simulink model "arducopter"  (R2021a)
settings: Solver=FixedStepAuto  StartTime=0.0  StopTime=sim.param.timeEnd  FixedStep=sim.param.dt  RelTol=1e-3
undefined symbols (not defined in the file or in its folder): DiscIntNeverNeededParam, sim
libraries: simulink x34, slident x4, vrlib x1
(part 7 of 8)

== matlab function arducopter/Position Controller/P Position z/Set vertical speed & acceleration limit/Set error limits ==
function [errMin, errMax, D1max] = setLimits(outMin, outMax, DoutMax, D2OutMax, kp)
% Code taken from AC_P_1D::set_limits() in AC_P_1D.cpp.
% Input parameter D2_out_max is neglected since it is set to zero in
% AC_PosControl::set_correction_speed_accel_z()

errMin = single(0.0);
errMax = single(0.0);
D1max = single(0.0);

if (DoutMax > 0)
   D1max = DoutMax; 
end

% Missing line left out because of parameter D2_out_max being set to 0

% Call the simulink function inv_sqrt_controller(...) from control.cpp,
% line 343 if the conditions apply
if (outMin < 0 && kp > 0)
    errMin = inv_sqrt_controller(outMin, kp, DoutMax);
end

if (outMax > 0 && kp > 0)
    errMax = inv_sqrt_controller(outMax, kp, DoutMax);
end

== matlab function arducopter/Position Controller/P Position z/Set vertical speed & acceleration limit/Inverse Square Root Controller/Inverse Sqrt Controller ==
function errLim = inv_sqrt_controller(output, p, Dmax)
% Code taken from inv_sqrt_controller(...) in control.cpp.
% Function calculates the input (error) to the sqrt_controller required to
% achieve a given output

if (Dmax > 0 && p == 0)
    errLim = output * output / (single(2.0) * Dmax);
    return;
end
if ((Dmax < 0 || Dmax == 0) && p ~= 0)
    errLim = output / p;
    return;
end
if ((Dmax < 0 || Dmax == 0) && p == 0)
   errLim = single(0.0);
   return
end

% Calculate the cross-point velocity, at which we switch from calculating the
% controller output using a linear function to a sqrt function
linear_velocity = Dmax / p;
% Use linear function to calculate limit if current velocity is below
% cross-point velocity
if (abs(output) < linear_velocity)
   errLim = output / p;
   return;
end

% Calculate the cross-point distance at which we switch to sqrt function
linear_dist = Dmax / (p*p);
% Calculate the maximum distance error resulting from the velocity and
% acceleration limit
stopping_dist = (linear_dist * single(0.5)) + (output*output) / (single(2.0) * Dmax);
% If output parameter is negative or zero, return negative maximum distance
% error
if (output > 0)
    errLim = stopping_dist;
else
    errLim = -stopping_dist;
end

== matlab function arducopter/Position Controller/P Position z/Square Root Controller ==
function correction_rate = sqrt_controller(err, p, second_ord_lim, dt)
% The square root controller
% Code is taken from sqrt_controller(...) in AC_PosControl.cpp.

if (second_ord_lim < 0 || second_ord_lim == 0)
   correction_rate = err * p;
elseif (p == 0)
    % P term is zero, but second order limit is positive
    if (err > 0)
        correction_rate = sqrt(single(2.0) * second_ord_lim * err);
    elseif (err < 0)
        correction_rate = sqrt(single(2.0) * second_ord_lim * -err);
    else
        correction_rate = single(0.0);
    end
else
    % P term and second order limit are positive, hence have been defined
    linear_dist = second_ord_lim / (p * p);
    % Check if error exceeds linear range of controller gain
    if (err > linear_dist)
        correction_rate = sqrt(single(2.0) * second_ord_lim * ( err - (linear_dist / single(2.0)) ));
    elseif (err < -linear_dist)
        correction_rate = -sqrt(single(2.0) * second_ord_lim * ( -err - (linear_dist / single(2.0)) ));
    else
        % Return linearly amplified correction if error is in linear range
        correction_rate = err * p;
    end
end

% Prevent oscillations by over-shooting the error correction in the last
% time step
if (dt ~= 0)
    correction_rate = max( min(correction_rate, abs(err) / dt), -abs(err) / dt);
end

== matlab function arducopter/Position Controller/PID Acceleration z/Slew Limiter/Lowpass Filter ==
function out  = fcn(in, cutoff_freq, loop_rate, out_last)
% The code is based on the apply(sample, cutoff_freq, dt) function in
% LowPassFilter.cpp
dt = 1 / loop_rate;

% Check if filter is supposed to be filtering
if (cutoff_freq <=0 || dt <= 0)
    out = in;
    return;
end

% Calculate time constant and alpha value
T = 1 / (2 * pi * cutoff_freq);
alpha = dt / (dt + T);
alpha = max( min( alpha, 1.0), 0.0);

% Output calculation
out = out_last + (in - out_last) * alpha;

== matlab function arducopter/Throttle/Throttle Calculations/Throttle-Attitude-Mixing/Update Throttle Mix Des ==
function thrMixDes = updateThrottleMix(thrTar, zVelCtrlRatio, zVelDes, thrMan, thrMixMin, thrMixMax, thrMixMan)
% Sets desired throttle vs attitude priorization based on vehicle state.
% Low values favour pilot/autpilot throttle over attitude control, high
% values favour attitude control over throttle
% Has not effec twhen throttle > hover throttle
% Code: land_detector.cpp, Copter::update_throttle_mix()

if thrMan
    % Manual throttle
    if thrTar <= 0
        % Call to set_throttle_mix_min() set mix to minimum
        thrMixDes = thrMixMin;
    else
        % Call to set_throttle_mix_man() sets mix to value for manual
        % throttle
        thrMixDes = thrMixMan;
    end
else
    % Autopilot controlled throttle
    
    % Check for aggressive flight request - Requested roll/pitch angle
    % above 15 degrees
    % ToDo

    % Check for large external disturbances - angle error over 30 degrees
    % ToDo

    % Check for large acceleration - falling for high turbulence
    % ToDo

    % Check for requested descent
    descent_not_demanded = zVelDes >= single(0.0);

    if (descent_not_demanded)
        % Call to AC_AttitudeControl_Multi::set_throttle_mix_max(ratio)
        ratio = min( max(single(0.0), zVelCtrlRatio), single(1.0) );
        thrMixDes = (single(1.0) - ratio) * thrMixMin + ratio * thrMixMax;
    else
        thrMixDes = thrMixMin;
    end
end

== matlab function arducopter/Position Controller/zVelCtrlRatio Calculation/Update vel_z_ctrl_ratio ==
function zVelCtrlRat = setZVelCtrlRatio(velErr, dnVelMax, dt)
% Sets vel_z_control_ratio, which contains the proportion of the z velocity
% error relative to the maximum request. Needed in function
% Copter::update_throttle_mix().
% Code: AC_PosControl.cpp, update_z_controller()

global vel_z_ctrl_ratio;

err_ratio = velErr / dnVelMax;
vel_z_ctrl_ratio = vel_z_ctrl_ratio + dt * single(0.1) * (0.5 - err_ratio);
vel_z_ctrl_ratio = min( max(single(0.0), vel_z_ctrl_ratio), single(2.0) );

zVelCtrlRat = vel_z_ctrl_ratio;

== matlab function arducopter/Position Controller/Vertical Speed and Acceleration Limits ==
function setMaxSpeedAccelZ(dnSpeedMax, upSpeedMax, zAccMax, zJerkMax, GRAVITY_MSS, zAccFltt_f, zAccFlte_f)
% Sets the maximum vertical speed in cm/s and acceleration in cm/s/s.
% Checks max vertical jerk limits.
% Code: AC_PosControl.cpp, set_max_speed_accel_z().

global vel_max_down_cms;
global vel_max_up_cms;
global acc_max_z_cmss;
global jerk_max_z_cmsss;

% Make sure maximum descending speed is negative
dnSpeedMax = dnSpeedMax * single(-1);

% Sanity check
if dnSpeedMax < 0
    vel_max_down_cms = dnSpeedMax;
end
if upSpeedMax > 0
    vel_max_up_cms = upSpeedMax;
end
if zAccMax > 0
    acc_max_z_cmss = zAccMax;
end

% Ensure that vertical jerk is not limited by filter of z acceleration PID
jerk_max_z_cmsss = single(100) * zJerkMax;
if (zAccFltt_f > 0)
    jerk_max_z_cmsss = min( jerk_max_z_cmsss, min(GRAVITY_MSS * single(100), acc_max_z_cmss) * (2*pi*zAccFltt_f) / single(5.0) );
end
if (zAccFlte_f > 0)
    jerk_max_z_cmsss = min( jerk_max_z_cmsss, min(GRAVITY_MSS * single(100), acc_max_z_cmss) * (2*pi*zAccFlte_f) / single(5.0) );
end

== matlab function arducopter/Lowpass2p/Lowpass Pitch/Lowpass2p ==
function y = lowpass2p(u, sampleFreq, cutoffFreq)
% Lowpass filter of order two
% Source: LowPassFilter2p.cpp
global delElem1
global delElem2

% Calculate parameters: LowPassFilter2p.cpp, compute_params()
fr = single(sampleFreq/cutoffFreq);
ohm = single(tan(pi/fr));
c = single(1+2*cos(pi/4)*ohm + ohm*ohm);

b0 = ohm*ohm/c;
b1 = 2*b0;
b2 = b0;
a1 = 2*(ohm*ohm-1)/c;
a2 = single((1-2*cos(pi/4)*ohm+ohm*ohm)/c);

% Calculation of filtered sample: LowPassFilter2p.cpp, apply()
delElem0 = u - delElem1 * a1 - delElem2 * a2;
y = delElem0 * b0 + delElem1 * b1 + delElem2 * b2;

delElem2 = delElem1;
delElem1 = delElem0;

== matlab function arducopter/Lowpass2p/Lowpass Roll/Lowpass2p ==
function y = lowpass2p(u, sampleFreq, cutoffFreq)
% Lowpass filter of order two
% Source: LowPassFilter2p.cpp
global delElem1
global delElem2

% Calculate parameters: LowPassFilter2p.cpp, compute_params()
fr = single(sampleFreq/cutoffFreq);
ohm = single(tan(pi/fr));
c = single(1+2*cos(pi/4)*ohm + ohm*ohm);

b0 = ohm*ohm/c;
b1 = 2*b0;
b2 = b0;
a1 = 2*(ohm*ohm-1)/c;
a2 = single((1-2*cos(pi/4)*ohm+ohm*ohm)/c);

% Calculation of filtered sample: LowPassFilter2p.cpp, apply()
delElem0 = u - delElem1 * a1 - delElem2 * a2;
y = delElem0 * b0 + delElem1 * b1 + delElem2 * b2;

delElem2 = delElem1;
delElem1 = delElem0;

== matlab function arducopter/Lowpass2p/Lowpass Yaw/Lowpass2p ==
function y = lowpass2p(u, sampleFreq, cutoffFreq)
% Lowpass filter of order two
% Source: LowPassFilter2p.cpp
global delElem1
global delElem2

% Calculate parameters: LowPassFilter2p.cpp, compute_params()
fr = single(sampleFreq/cutoffFreq);
ohm = single(tan(pi/fr));
c = single(1+2*cos(pi/4)*ohm + ohm*ohm);

b0 = ohm*ohm/c;
b1 = 2*b0;
b2 = b0;
a1 = 2*(ohm*ohm-1)/c;
a2 = single((1-2*cos(pi/4)*ohm+ohm*ohm)/c);

% Calculation of filtered sample: LowPassFilter2p.cpp, apply()
delElem0 = u - delElem1 * a1 - delElem2 * a2;
y = delElem0 * b0 + delElem1 * b1 + delElem2 * b2;

delElem2 = delElem1;
delElem1 = delElem0;

== matlab function arducopter/Body Frame Rates -> DCM/MATLAB Function ==
function quaternion = from_rotation_matrix(dcm)
% Function to calculate quaternion from a given rotation matrix.
% Implemented based on QuaternionT<T>::from_rotation_matrx()

m00 = dcm(1,1);
m11 = dcm(2,2);
m22 = dcm(3,3);
m10 = dcm(2,1);
m01 = dcm(1,2);
m20 = dcm(3,1);
m02 = dcm(1,3);
m21 = dcm(3,2);
m12 = dcm(2,3);

tr = m00 + m11 + m22;

if tr > 0
    S = sqrt(tr+1) * 2;
    qw = 0.25 * S;
    qx = (m21 - m12) / S;
    qy = (m02 - m20) / S;
    qz = (m10 - m01) / S;
elseif ((m00 > m11) && (m00 > m22))
    S = sqrt(1.0 + m00 - m11 - m22) * 2.0;
    qw = (m21 - m12) / S;
    qx = 0.25 * S;
    qy = (m01 + m10) / S;
    qz = (m02 + m20) / S;
elseif (m11 > m22)
    S = sqrt(1.0 + m11 - m00 - m22) * 2.0;
    qw = (m02 - m20) / S;
    qx = (m01 + m10) / S;
    qy = 0.25 * S;
    qz = (m12 + m21) / S;
else
    S = sqrt(1.0 + m22 - m00 - m11) * 2.0;
    qw = (m10 - m01) / S;
    qx = (m02 + m20) / S;
    qy = (m12 + m21) / S;
    qz = 0.25 * S;
end

quaternion = [qw;qx;qy;qz];

== matlab function arducopter/Attitude Controller/MATLAB Function ==
function [rollOut, pitchOut] = get_pilot_desired_lean_angles(rollIn, pitchIn, angleMax, angleLimit)
% Code based on Mode::get_pilot_desired_lean_angles()
% Transform pilot's roll and pitch input into desired lean angle

% Limit max lean angle
angleLimit = max(min(angleLimit, angleMax), 1000);

% Scale roll and pitch inputs to ANGLE_MAX parameter range
scaler = angleMax / 4500; % 4500 is the default of ROLL_PITCH_YAW_INPUT_MAX
rollOut = rollIn * scaler;
pitchOut = pitchIn * scaler;

% Circular limit
quadNorm = sqrt(rollOut^2 + pitchOut^2);
if quadNorm > angleLimit
    ratio = angleLimit / quadNorm;
    rollOut = rollOut * ratio;
    pitchOut = pitchOut * ratio;
end

% Lateral tilt to euler roll conversion
rollOut = (18000/pi) * atan(cos(pitchOut*(pi/18000))*tan(rollOut*(pi/18000)));

== matlab function arducopter/Attitude Controller/MATLAB Function1 ==
function yawOut = get_pilot_desired_yaw_rate(yawIn, pilotYawExpo, pilotYawRate)
% Code taken from Mode::get_pilot_desired_yaw_rate()
% Transforms pilot's yaw input into a desired yaw rate

%% 1) Apply expo - Code based on input_expo in control.cpp
yawIn = min(max(yawIn, -1), 1);
if pilotYawExpo < 0.95
    yawIn = (1 - pilotYawExpo) * yawIn / (1 - pilotYawExpo * abs(yawIn));
end

%% 2) Convert pilot input to the desired yaw rate
yawOut = pilotYawRate * 100 * yawIn;

== matlab function arducopter/Attitude Controller/input_euler_angle_roll_pitch_euler_rate_yaw()/MATLAB Function ==
function [roll, pitch, yaw] = toEuler(q)
% Function takes a quaternion and translates it into Euler angles
% Based on QuaternionT<T>::to_euler() and incorporates 
% QuaternionT<T>::get_euler_roll(), QuaternionT<T>::get_euler_pitch() and
% QuaternionT<T>::get_euler_yaw()

roll = single(atan2(2 * (q(1)*q(2) + q(3)*q(4)), 1 - 2*(q(2)*q(2) + q(3)*q(3))));
% Check if argument of asin is greater than 1 oder smaller than -1
% Based on safe_asin() in AP_MATH.cpp
xPitch = 2 * (q(1)*q(3) - q(4)*q(2));
if xPitch >= 1
    pitch = single(pi/2);
elseif xPitch <= -1
    pitch = single(-pi/2);
else
    pitch = single(asin(xPitch));
end
yaw = single(atan2(2*(q(1)*q(4) + q(2)*q(3)), 1 - 2*(q(3)*q(3) + q(4)*q(4))));

== matlab function arducopter/Attitude Controller/input_euler_angle_roll_pitch_euler_rate_yaw()/Feedforward enabled/MATLAB Function ==
function eulerAccelMaxBF = euler_accel_limit(eulerAngleTar, eulerAccelMaxEF)
% Translation of acceleration limits eulerAccelMax to the euler axis
% Code based on AC_AttitudeControl::euler_accel_limit()

sin_phi = max(min(abs(single(sin(eulerAngleTar(1)))), 1), 0.1); % Sinus of roll angle
cos_phi = max(min(abs(single(cos(eulerAngleTar(1)))), 1), 0.1);
sin_theta = max(min(abs(single(sin(eulerAngleTar(2)))), 1), 0.1); % Sinus of pitch angle

eulerAccelMaxBF = single(zeros(3,1));
if eulerAccelMaxEF(1) == 0 || eulerAccelMaxEF(2) == 0 || eulerAccelMaxEF(3) == 0 || ...
   eulerAccelMaxEF(1) < 0 || eulerAccelMaxEF(2) < 0 || eulerAccelMaxEF(3) < 0 
    eulerAccelMaxBF(1) = eulerAccelMaxEF(1);
    eulerAccelMaxBF(2) = eulerAccelMaxEF(2);
    eulerAccelMaxBF(3) = eulerAccelMaxEF(3);
else
    eulerAccelMaxBF(1) = eulerAccelMaxEF(1);
    eulerAccelMaxBF(2) = min(eulerAccelMaxEF(2) / cos_phi, eulerAccelMaxEF(3) / sin_phi);
    eulerAccelMaxBF(3) = min(min(eulerAccelMaxEF(1) / sin_theta, eulerAccelMaxEF(2) / sin_phi), eulerAccelMaxEF(3) / cos_phi);
end

== matlab function arducopter/Attitude Controller/input_euler_angle_roll_pitch_euler_rate_yaw()/Feedforward enabled/input shaping/input shaping roll angle/Square Root Controller ==
function correction_rate = sqrt_controller(err, p, second_ord_lim, dt)
% The square root controller
% Code is taken from sqrt_controller(...) in AC_PosControl.cpp, line 296.

if (second_ord_lim < 0 || second_ord_lim == 0)
   correction_rate = err * p;
elseif (p == 0)
    % P term is zero, but second order limit is positive
    if (err > 0)
        correction_rate = sqrt(single(2.0) * second_ord_lim * err);
    elseif (err < 0)
        correction_rate = sqrt(single(2.0) * second_ord_lim * -err);
    else
        correction_rate = single(0.0);
    end
else
    % P term and second order limit are positive, hence have been defined
    linear_dist = second_ord_lim / (p * p);
    % Check if error exceeds linear range of controller gain
    if (err > linear_dist)
        correction_rate = sqrt(single(2.0) * second_ord_lim * ( err - (linear_dist / single(2.0)) ));
    elseif (err < -linear_dist)
        correction_rate = -sqrt(single(2.0) * second_ord_lim * ( -err - (linear_dist / single(2.0)) ));
    else
        % Return linearly amplified correction if error is in linear range
        correction_rate = err * p;
    end
end

% Prevent oscillations by over-shooting the error correction in the last
% time step
if (dt ~= 0)
    correction_rate = max( min(correction_rate, abs(err) / dt), -abs(err) / dt);
end

== matlab function arducopter/Attitude Controller/input_euler_angle_roll_pitch_euler_rate_yaw()/Feedforward enabled/input shaping/input shaping roll angle/MATLAB Function ==
function radLim = wrapPi(radIn)
% Function to limit input angle in radian to [-pi pi].
% Code based on wrap_PI() and wrap_2PI() of AP_Math.cpp

% 1) Limit to [0 2pi]
radLim = mod(radIn, 2*pi);
if radLim < 0
    radLim = radLim + 2*pi;
end

% 2) Limit to [0 pi]
if radLim > pi
    radLim = radLim - 2*pi;
end

== matlab function arducopter/Attitude Controller/input_euler_angle_roll_pitch_euler_rate_yaw()/Feedforward enabled/input shaping/input shaping roll angle/MATLAB Function1 ==
function eulerRateTar = input_shaping_ang_vel(desiredAngVel, targetAngVel, accelMax, dt)
% Limits acceleration and deceleration of a velocity request
% Code based on AC_AttitudeControl::input_shaping_ang_vel()

% Acceleration is limited directly to smooth the beginning of the curve
if accelMax > 0
    deltaAngVel = accelMax * dt;
    eulerRateTar = min(max(desiredAngVel, targetAngVel - deltaAngVel), targetAngVel + deltaAngVel);
else
    eulerRateTar = desiredAngVel;
end

== matlab function arducopter/Attitude Controller/input_euler_angle_roll_pitch_euler_rate_yaw()/Feedforward enabled/input shaping/input shaping pitch angle/MATLAB Function ==
function radLim = wrapPi(radIn)
% Function to limit input angle in radian to [-pi pi].
% Code based on wrap_PI() and wrap_2PI() of AP_Math.cpp

% 1) Limit to [0 2pi]
radLim = mod(radIn, 2*pi);
if radLim < 0
    radLim = radLim + 2*pi;
end

% 2) Limit to [0 pi]
if radLim > pi
    radLim = radLim - 2*pi;
end

== matlab function arducopter/Attitude Controller/input_euler_angle_roll_pitch_euler_rate_yaw()/reset yaw targets/MATLAB Function9 ==
function qRes = quatMult(q1, q2)
% Quaternion multiplication. Code based on QuaternionT<T>::operator*() in
% quaternion.cpp

qRes = single(zeros(4,1));
qRes(1) = q1(1)*q2(1) - q1(2)*q2(2) - q1(3)*q2(3) - q1(4)*q2(4);
qRes(2) = q1(1)*q2(2) + q1(2)*q2(1) + q1(3)*q2(4) - q1(4)*q2(3);
qRes(3) = q1(1)*q2(3) - q1(2)*q2(4) + q1(3)*q2(1) + q1(4)*q2(2);
qRes(4) = q1(1)*q2(4) + q1(2)*q2(3) - q1(3)*q2(2) + q1(4)*q2(1);

== matlab function arducopter/Attitude Controller/input_euler_angle_roll_pitch_euler_rate_yaw()/Feedforward enabled/input shaping/input shaping pitch angle/Square Root Controller ==
function correction_rate = sqrt_controller(err, p, second_ord_lim, dt)
% The square root controller
% Code is taken from sqrt_controller(...) in AC_PosControl.cpp, line 296.

if (second_ord_lim < 0 || second_ord_lim == 0)
   correction_rate = err * p;
elseif (p == 0)
    % P term is zero, but second order limit is positive
    if (err > 0)
        correction_rate = sqrt(single(2.0) * second_ord_lim * err);
    elseif (err < 0)
        correction_rate = sqrt(single(2.0) * second_ord_lim * -err);
    else
        correction_rate = single(0.0);
    end
else
    % P term and second order limit are positive, hence have been defined
    linear_dist = second_ord_lim / (p * p);
    % Check if error exceeds linear range of controller gain
    if (err > linear_dist)
        correction_rate = sqrt(single(2.0) * second_ord_lim * ( err - (linear_dist / single(2.0)) ));
    elseif (err < -linear_dist)
        correction_rate = -sqrt(single(2.0) * second_ord_lim * ( -err - (linear_dist / single(2.0)) ));
    else
        % Return linearly amplified correction if error is in linear range
        correction_rate = err * p;
    end
end

% Prevent oscillations by over-shooting the error correction in the last
% time step
if (dt ~= 0)
    correction_rate = max( min(correction_rate, abs(err) / dt), -abs(err) / dt);
end

== matlab function arducopter/Attitude Controller/input_euler_angle_roll_pitch_euler_rate_yaw()/Feedforward enabled/MATLAB Function1 ==
function angVelTar = euler_rate_to_ang_vel(eulerAngle, eulerRate)
% This function converts euler angle derivatives (321 system) to an angular
% velocity vector. eulerAngle is the vector of the euler angles in rad and
% eulerRate is the vector of euler rates in rad/s
% Code based on AC_AttitudeControl::euler_rate_to_ang_vel()

sin_theta = single(sin(eulerAngle(2)));
cos_theta = single(cos(eulerAngle(2)));
sin_phi = single(sin(eulerAngle(1)));
cos_phi = single(cos(eulerAngle(1)));

angVelTar = single(zeros(3,1));
angVelTar(1) = eulerRate(1) - sin_theta * eulerRate(3);
angVelTar(2) = cos_phi * eulerRate(2) + sin_phi * cos_theta * eulerRate(3);
angVelTar(3) = -sin_phi * eulerRate(2) + cos_theta * cos_phi * eulerRate(3);

== matlab function arducopter/Rate Controller/PID Pitch Rate/I/Integrator ==
function integrator_out = fcn(error, integrator, limit_flg, ki, i_max, dt)
% Code is based on AC_PID::update_i() in AC_PID.cpp.

% Check plausibility of input parameters
if (ki ~= 0 && dt > 0)
    % Only allow integration if limit is not set or the absolute sum of the
    % integrator would be reduced.
    if (~limit_flg || (integrator > 0 && error < 0) || (integrator < 0 && error > 0))
        integrator_out = integrator + error * ki * dt;
        integrator_out = max( min(integrator_out, i_max), -i_max);
    else % Otherwise, keep old integrator value
        integrator_out = integrator;
    end
else % Reset integrator if input parameters are not plausible
    integrator_out = single(0.0);
end

== matlab function arducopter/Attitude Controller/input_euler_angle_roll_pitch_euler_rate_yaw()/reset yaw targets/MATLAB Function1 ==
function [roll, pitch, yaw] = toEuler(q)
% Function takes a quaternion and translates it into Euler angles
% Based on QuaternionT<T>::to_euler() and incorporates 
% QuaternionT<T>::get_euler_roll(), QuaternionT<T>::get_euler_pitch() and
% QuaternionT<T>::get_euler_yaw()

roll = single(atan2(2 * (q(1)*q(2) + q(3)*q(4)), 1 - 2*(q(2)*q(2) + q(3)*q(3))));
% Check if argument of asin is greater than 1 oder smaller than -1
% Based on safe_asin() in AP_MATH.cpp
xPitch = 2 * (q(1)*q(3) - q(4)*q(2));
if xPitch >= 1
    pitch = single(pi/2);
elseif xPitch <= -1
    pitch = single(-pi/2);
else
    pitch = single(asin(xPitch));
end
yaw = single(atan2(2*(q(1)*q(4) + q(2)*q(3)), 1 - 2*(q(3)*q(3) + q(4)*q(4))));

== matlab function arducopter/Attitude Controller/input_euler_angle_roll_pitch_euler_rate_yaw()/Feedforward enabled/MATLAB Function2 ==
function angVelTarLimited = ang_vel_limit(angVelTar, angVelRollMax, angVelPitchMax, angVelYawMax)
% Limits angular velocity (rad/s) in body frame
% Code based on AC_AttitudeControl::ang_vel_limit()

angVelTarLimited = angVelTar;
if angVelRollMax == 0 || angVelPitchMax == 0
    if angVelRollMax ~= 0
        angVelTarLimited(1) = max(min(angVelTar(1), angVelRollMax), -angVelRollMax);
    end
    if angVelPitchMax ~= 0
        angVelTarLimited(2) = max(min(angVelTar(2), angVelPitchMax), -angVelPitchMax);
    end
else
    thrustVecAngVel = [angVelTar(1) / angVelRollMax; angVelTar(2) / angVelPitchMax];
    thrustVecLen = single(sqrt(thrustVecAngVel(1)^2 + thrustVecAngVel(2)^2));
    if thrustVecLen > 1
        angVelTarLimited(1) = thrustVecAngVel(1) * angVelRollMax / thrustVecLen;
        angVelTarLimited(2) = thrustVecAngVel(2) * angVelPitchMax / thrustVecLen;
    end
end
if angVelYawMax ~= 0
    angVelTarLimited(3) = max(min(angVelTar(3), angVelYawMax), -angVelYawMax);
end

== matlab function arducopter/Attitude Controller/input_euler_angle_roll_pitch_euler_rate_yaw()/Feedforward enabled/MATLAB Function3 ==
function eulerRate = ang_vel_to_euler_rate(angVelBf,eulerAngle)
% Function converts body-frame angular velocity into euler rate of desired
% attitude
% Based on AC_AttitudeControl::ang_vel_to_euler_rate()

sin_theta = single(sin(eulerAngle(2)));
cos_theta = single(cos(eulerAngle(2)));
sin_phi = single(sin(eulerAngle(1)));
cos_phi = single(cos(eulerAngle(1)));

eulerRate = single(zeros(3,1));
eulerRate(1) = angVelBf(1) + sin_phi * (sin_theta / cos_theta) * angVelBf(2) + cos_phi * (sin_theta / cos_theta) * angVelBf(3);
eulerRate(2) = cos_phi * angVelBf(2) - sin_phi * angVelBf(3);
eulerRate(3) = (sin_phi / cos_theta) * angVelBf(2) + (cos_phi / cos_theta) * angVelBf(3);

== matlab function arducopter/Attitude Controller/input_euler_angle_roll_pitch_euler_rate_yaw()/Feedforward disabled/MATLAB Function ==
function q = fromEuler(roll, pitch, yaw)
% Computes quaternion from euler angle vector
% Based on QuaternionT<T>::from_euler()

q = single(zeros(4,1));
cr2 = single(cos(roll*0.5));
cp2 = single(cos(pitch*0.5));
cy2 = single(cos(yaw*0.5));
sr2 = single(sin(roll*0.5));
sp2 = single(sin(pitch*0.5));
sy2 = single(sin(yaw*0.5));

q(1) = cr2*cp2*cy2 + sr2*sp2*sy2;
q(2) = sr2*cp2*cy2 - cr2*sp2*sy2;
q(3) = cr2*sp2*cy2 + sr2*cp2*sy2;
q(4) = cr2*cp2*sy2 - sr2*sp2*cy2;

== matlab function arducopter/Attitude Controller/input_euler_angle_roll_pitch_euler_rate_yaw()/thrust_heading_rotation_angles()/thrust_vector_rotation_angles()/MATLAB Function ==
function vecRot = rotateByQuat(q, vec)
% Function rotates vector vec by quaternion q. Equivalent to converting the
% input quaternion to a rotation matrix and then multiplying it by the
% vector. This uses the formula
%
%    v2 = v1 + 2 q1 * qv x v1 + 2 qv x qv x v1
%
% where "x" is the cross product (explicitly inlined for performance below), 
% "q1" is the scalar part and "qv" is the vector part of this quaternion
% Code based on Vector3<T> QuaternionT<T>::operator*()

vecRot = vec;

% Compute and cache "qv x v1"
uv = [q(3) * vec(3) - q(4) * vec(2); q(4) * vec(1) - q(2) * vec(3); q(2) * vec(2) - q(3) * vec(1)];

uv(1) = uv(1) + uv(1);
uv(2) = uv(2) + uv(2);
uv(3) = uv(3) + uv(3);
vecRot(1) = vecRot(1) + q(1) * uv(1) + q(3) * uv(3) - q(4) * uv(2);
vecRot(2) = vecRot(2) + q(1) * uv(2) + q(4) * uv(1) - q(2) * uv(3);
vecRot(3) = vecRot(3) + q(1) * uv(3) + q(2) * uv(2) - q(3) * uv(1);

== matlab function arducopter/Attitude Controller/input_euler_angle_roll_pitch_euler_rate_yaw()/thrust_heading_rotation_angles()/thrust_vector_rotation_angles()/MATLAB Function1 ==
function vecRot = rotateByQuat(q, vec)
% Function rotates vector vec by quaternion q. Equivalent to converting the
% input quaternion to a rotation matrix and then multiplying it by the
% vector. This uses the formula
%
%    v2 = v1 + 2 q1 * qv x v1 + 2 qv x qv x v1
%
% where "x" is the cross product (explicitly inlined for performance below), 
% "q1" is the scalar part and "qv" is the vector part of this quaternion
% Code based on Vector3<T> QuaternionT<T>::operator*()

vecRot = vec;

% Compute and cache "qv x v1"
uv = [q(3) * vec(3) - q(4) * vec(2); q(4) * vec(1) - q(2) * vec(3); q(2) * vec(2) - q(3) * vec(1)];

uv(1) = uv(1) + uv(1);
uv(2) = uv(2) + uv(2);
uv(3) = uv(3) + uv(3);
vecRot(1) = vecRot(1) + q(1) * uv(1) + q(3) * uv(3) - q(4) * uv(2);
vecRot(2) = vecRot(2) + q(1) * uv(2) + q(4) * uv(1) - q(2) * uv(3);
vecRot(3) = vecRot(3) + q(1) * uv(3) + q(2) * uv(2) - q(3) * uv(1);

== matlab function arducopter/Attitude Controller/input_euler_angle_roll_pitch_euler_rate_yaw()/thrust_heading_rotation_angles()/thrust_vector_rotation_angles()/MATLAB Function2 ==
function rotVecNorm = normalizeVec(thrustErrAngle, rotVec)
% Function to normalize the thrust rotation vector. Divides the vector by
% its length or uses up-vector if thrust error angle is zero
rotVecNorm = single(zeros(3,1));
vecLen = single(sqrt(rotVec(1)^2 + rotVec(2)^2 + rotVec(3)^2));

if thrustErrAngle == 0 || vecLen == 0
    rotVecNorm = single([0;0;-1]);
else
    rotVecNorm(1) = rotVec(1) / vecLen;
    rotVecNorm(2) = rotVec(2) / vecLen;
    rotVecNorm(3) = rotVec(3) / vecLen;
end

== matlab function arducopter/Attitude Controller/input_euler_angle_roll_pitch_euler_rate_yaw()/thrust_heading_rotation_angles()/thrust_vector_rotation_angles()/MATLAB Function3 ==
function qInv = invertQuat(q)
% Function inverts the rotation of a quaternion.
% Code based on QuaternionT<T>::inverse(void)
% qInv = [q(1);-q(2);-q(3);-q(4)];
qInv = single(zeros(4,1));
qInv(1) = q(1);
qInv(2) = -q(2);
qInv(3) = -q(3);
qInv(4) = -q(4);

== matlab function arducopter/Attitude Controller/input_euler_angle_roll_pitch_euler_rate_yaw()/thrust_heading_rotation_angles()/thrust_vector_rotation_angles()/MATLAB Function4 ==
function vecRot = rotateByQuat(q, vec)
% Function rotates vector vec by quaternion q. Equivalent to converting the
% input quaternion to a rotation matrix and then multiplying it by the
% vector. This uses the formula
%
%    v2 = v1 + 2 q1 * qv x v1 + 2 qv x qv x v1
%
% where "x" is the cross product (explicitly inlined for performance below), 
% "q1" is the scalar part and "qv" is the vector part of this quaternion
% Code based on Vector3<T> QuaternionT<T>::operator*()

vecRot = vec;

% Compute and cache "qv x v1"
uv = [q(3) * vec(3) - q(4) * vec(2); q(4) * vec(1) - q(2) * vec(3); q(2) * vec(2) - q(3) * vec(1)];

uv(1) = uv(1) + uv(1);
uv(2) = uv(2) + uv(2);
uv(3) = uv(3) + uv(3);
vecRot(1) = vecRot(1) + q(1) * uv(1) + q(3) * uv(3) - q(4) * uv(2);
vecRot(2) = vecRot(2) + q(1) * uv(2) + q(4) * uv(1) - q(2) * uv(3);
vecRot(3) = vecRot(3) + q(1) * uv(3) + q(2) * uv(2) - q(3) * uv(1);

== matlab function arducopter/Attitude Controller/input_euler_angle_roll_pitch_euler_rate_yaw()/thrust_heading_rotation_angles()/thrust_vector_rotation_angles()/MATLAB Function5 ==
function q = fromAxisAngle(axis, angle)
% Create a quaternion from its axis-angle representation. The axis-vector
% must be of length 1 and the angle in radians.
% Based on QuaternionT<T>::from_axis_angle()

q = single(zeros(4,1));

if angle == 0
    q(1) = 1;
    q(2) = 0;
    q(3) = 0;
    q(4) = 0;
else
    st2 = sin(0.5*angle);
    q(1) = cos(0.5*angle);
    q(2) = axis(1) * st2;
    q(3) = axis(2) * st2;
    q(4) = axis(3) * st2;
end

== matlab function arducopter/Attitude Controller/input_euler_angle_roll_pitch_euler_rate_yaw()/thrust_heading_rotation_angles()/thrust_vector_rotation_angles()/MATLAB Function6 ==
function vec = toAxisAngle(q)
% Converts the quaternion to a rotation vector. The direction represents
% the axis of rotation and the length represents the angle of rotation
% Code based on QuaternionT<T>::to_axis_angle()
l = sqrt(q(2)^2 + q(3)^2 + q(4)^2);

vec = [q(2);q(3);q(4)];

if l ~= 0
    vec = vec ./ l;
    mult = 2 * atan2(l, q(1));
    % The following lines are taken from wrap_pi() in AP_Math.cpp
    mult = mod(mult, 2*pi);
    if mult < 0
        mult = mult + 2*pi;
    end
    if mult > pi
        mult = mult - 2*pi;
    end

    vec = vec .* mult;
end

== matlab function arducopter/Attitude Controller/input_euler_angle_roll_pitch_euler_rate_yaw()/thrust_heading_rotation_angles()/thrust_vector_rotation_angles()/MATLAB Function7 ==
function qInv = invertQuat(q)
% Function inverts the rotation of a quaternion.
% Code based on QuaternionT<T>::inverse(void)
% qInv = [q(1);-q(2);-q(3);-q(4)];
qInv = single(zeros(4,1));
qInv(1) = q(1);
qInv(2) = -q(2);
qInv(3) = -q(3);
qInv(4) = -q(4);

== matlab function arducopter/Attitude Controller/input_euler_angle_roll_pitch_euler_rate_yaw()/thrust_heading_rotation_angles()/thrust_vector_rotation_angles()/MATLAB Function8 ==
function qInv = invertQuat(q)
% Function inverts the rotation of a quaternion.
% Code based on QuaternionT<T>::inverse(void)
qInv = [q(1);-q(2);-q(3);-q(4)];

== matlab function arducopter/Attitude Controller/input_euler_angle_roll_pitch_euler_rate_yaw()/thrust_heading_rotation_angles()/thrust_vector_rotation_angles()/MATLAB Function9 ==
function qRes = quatMult(q1, q2)
% Quaternion multiplication. Code based on QuaternionT<T>::operator*() in
% quaternion.cpp

qRes = single(zeros(4,1));
qRes(1) = q1(1)*q2(1) - q1(2)*q2(2) - q1(3)*q2(3) - q1(4)*q2(4);
qRes(2) = q1(1)*q2(2) + q1(2)*q2(1) + q1(3)*q2(4) - q1(4)*q2(3);
qRes(3) = q1(1)*q2(3) - q1(2)*q2(4) + q1(3)*q2(1) + q1(4)*q2(2);
qRes(4) = q1(1)*q2(4) + q1(2)*q2(3) - q1(3)*q2(2) + q1(4)*q2(1);

== matlab function arducopter/Attitude Controller/input_euler_angle_roll_pitch_euler_rate_yaw()/thrust_heading_rotation_angles()/thrust_vector_rotation_angles()/MATLAB Function10 ==
function vec = toAxisAngle(q)
% Converts the quaternion to a rotation vector. The direction represents
% the axis of rotation and the length represents the angle of rotation
% Code based on QuaternionT<T>::to_axis_angle()
l = sqrt(q(2)^2 + q(3)^2 + q(4)^2);

vec = [q(2);q(3);q(4)];

if l ~= 0
    vec = vec ./ l;
    mult = 2 * atan2(l, q(1));
    % The following lines are taken from wrap_pi() in AP_Math.cpp
    mult = mod(mult, 2*pi);
    if mult < 0
        mult = mult + 2*pi;
    end
    if mult > pi
        mult = mult - 2*pi;
    end

    vec = vec .* mult;
end

== matlab function arducopter/Throttle/Throttle Calculations/Boost and Premixing/Throttle_In Handling ==
function [thrOut, thrAvgMax] = fcn(thrTar, angBst, thrHover, angBstEna, thrRpyMix)
% The following lines represent the set_throttle_out() function in
% AC_AttitudeControl_Multi.cpp, that takes the desired throttle from the
% pilot and calculate the boosted and average max throttle.
if(angBstEna)
    % Reference: AC_AttitudeControl_Multi::get_throttle_boosted(throttle_in)
    thrOut = thrTar + angBst;
else
    thrOut = thrTar;
end

%% Determine throttle_avg_max
thr_des_max = max(thrOut, thrTar);

% The following lines are taken from get_throttle_avg_max()
% Limit throttle_max to [0,1]
thr_des_max = min( max( thr_des_max, 0), 1);

% Calculate maximum throttle between input throttle and needed throttle
% considering mix between roll/pitch and hovering
thrAvgMax = max(thr_des_max, thr_des_max * max( 0, (1-thrRpyMix) ) + thrHover * thrRpyMix);

== matlab function arducopter/Attitude Controller/input_euler_angle_roll_pitch_euler_rate_yaw()/thrust_heading_rotation_angles()/thrust_vector_rotation_angles()/MATLAB Function11 ==
function qRes = quatMult(q1, q2)
% Quaternion multiplication. Code based on QuaternionT<T>::operator*() in
% quaternion.cpp

qRes = single(zeros(4,1));
qRes(1) = q1(1)*q2(1) - q1(2)*q2(2) - q1(3)*q2(3) - q1(4)*q2(4);
qRes(2) = q1(1)*q2(2) + q1(2)*q2(1) + q1(3)*q2(4) - q1(4)*q2(3);
qRes(3) = q1(1)*q2(3) - q1(2)*q2(4) + q1(3)*q2(1) + q1(4)*q2(2);
qRes(4) = q1(1)*q2(4) + q1(2)*q2(3) - q1(3)*q2(2) + q1(4)*q2(1);

== matlab function arducopter/Attitude Controller/input_euler_angle_roll_pitch_euler_rate_yaw()/thrust_heading_rotation_angles()/thrust_vector_rotation_angles()/MATLAB Function12 ==
function qRes = quatMult(q1, q2)
% Quaternion multiplication. Code based on QuaternionT<T>::operator*() in
% quaternion.cpp

qRes = single(zeros(4,1));
qRes(1) = q1(1)*q2(1) - q1(2)*q2(2) - q1(3)*q2(3) - q1(4)*q2(4);
qRes(2) = q1(1)*q2(2) + q1(2)*q2(1) + q1(3)*q2(4) - q1(4)*q2(3);
qRes(3) = q1(1)*q2(3) - q1(2)*q2(4) + q1(3)*q2(1) + q1(4)*q2(2);
qRes(4) = q1(1)*q2(4) + q1(2)*q2(3) - q1(3)*q2(2) + q1(4)*q2(1);

== matlab function arducopter/Attitude Controller/input_euler_angle_roll_pitch_euler_rate_yaw()/thrust_heading_rotation_angles()/thrust_vector_rotation_angles()/MATLAB Function13 ==
function qInv = invertQuat(q)
% Function inverts the rotation of a quaternion.
% Code based on QuaternionT<T>::inverse(void)
qInv = [q(1);-q(2);-q(3);-q(4)];

== matlab function arducopter/Attitude Controller/input_euler_angle_roll_pitch_euler_rate_yaw()/thrust_heading_rotation_angles()/thrust_vector_rotation_angles()/MATLAB Function14 ==
function qInv = invertQuat(q)
% Function inverts the rotation of a quaternion.
% Code based on QuaternionT<T>::inverse(void)
qInv = [q(1);-q(2);-q(3);-q(4)];

== matlab function arducopter/Attitude Controller/input_euler_angle_roll_pitch_euler_rate_yaw()/thrust_heading_rotation_angles()/thrust_vector_rotation_angles()/MATLAB Function15 ==
function qRes = quatMult(q1, q2)
% Quaternion multiplication. Code based on QuaternionT<T>::operator*() in
% quaternion.cpp

qRes = single(zeros(4,1));
qRes(1) = q1(1)*q2(1) - q1(2)*q2(2) - q1(3)*q2(3) - q1(4)*q2(4);
qRes(2) = q1(1)*q2(2) + q1(2)*q2(1) + q1(3)*q2(4) - q1(4)*q2(3);
qRes(3) = q1(1)*q2(3) - q1(2)*q2(4) + q1(3)*q2(1) + q1(4)*q2(2);
qRes(4) = q1(1)*q2(4) + q1(2)*q2(3) - q1(3)*q2(2) + q1(4)*q2(1);

== matlab function arducopter/Attitude Controller/input_euler_angle_roll_pitch_euler_rate_yaw()/thrust_heading_rotation_angles()/thrust_vector_rotation_angles()/MATLAB Function16 ==
function vec = toAxisAngle(q)
% Converts the quaternion to a rotation vector. The direction represents
% the axis of rotation and the length represents the angle of rotation
% Code based on QuaternionT<T>::to_axis_angle()
l = sqrt(q(2)^2 + q(3)^2 + q(4)^2);

vec = [q(2);q(3);q(4)];

if l ~= 0
    vec = vec ./ l;
    mult = 2 * atan2(l, q(1));
    % The following lines are taken from wrap_pi() in AP_Math.cpp
    mult = mod(mult, 2*pi);
    if mult < 0
        mult = mult + 2*pi;
    end
    if mult > pi
        mult = mult - 2*pi;
    end

    vec = vec .* mult;
end

== matlab function arducopter/Attitude Controller/input_euler_angle_roll_pitch_euler_rate_yaw()/thrust_heading_rotation_angles()/Yaw error limitation/Yaw limiting and recalculation of attitudeTarget/MATLAB Function ==
function radLim = wrapPi(radIn)
% Function to limit input angle in radian to [-pi pi].
% Code based on wrap_PI() and wrap_2PI() of AP_Math.cpp

% 1) Limit to [0 2pi]
radLim = mod(radIn, 2*pi);
if radLim < 0
    radLim = radLim + 2*pi;
end

% 2) Limit to [0 pi]
if radLim > pi
    radLim = radLim - 2*pi;
end

== matlab function arducopter/Attitude Controller/input_euler_angle_roll_pitch_euler_rate_yaw()/thrust_heading_rotation_angles()/Yaw error limitation/Yaw limiting and recalculation of attitudeTarget/MATLAB Function5 ==
function q = fromAxisAngle(vec)
% Create a quaternion from its axis-angle representation. Just the rotation
% vector is given as input.
% Based on QuaternionT<T>::from_axis_angle(Vector3<T>)

q = single(zeros(4,1));
angle = sqrt(vec(1)^2 + vec(2)^2 + vec(3)^2);

if angle == 0
    q(1) = 1;
    q(2) = 0;
    q(3) = 0;
    q(4) = 0;
else
    axis = vec ./ angle;
    % The following lines are based on QuaternionT<T>::from_axis_angle(const Vector3<T> &axis, T theta)
    if angle == 0
        q(1) = 1;
        q(2) = 0;
        q(3) = 0;
        q(4) = 0;
    else
        st2 = sin(0.5*angle);
        q(1) = cos(0.5*angle);
        q(2) = axis(1) * st2;
        q(3) = axis(2) * st2;
        q(4) = axis(3) * st2;
    end
end

== matlab function arducopter/Attitude Controller/input_euler_angle_roll_pitch_euler_rate_yaw()/thrust_heading_rotation_angles()/Yaw error limitation/Yaw limiting and recalculation of attitudeTarget/MATLAB Function9 ==
function qRes = quatMult(q1, q2)
% Quaternion multiplication. Code based on QuaternionT<T>::operator*() in
% quaternion.cpp

qRes = single(zeros(4,1));
qRes(1) = q1(1)*q2(1) - q1(2)*q2(2) - q1(3)*q2(3) - q1(4)*q2(4);
qRes(2) = q1(1)*q2(2) + q1(2)*q2(1) + q1(3)*q2(4) - q1(4)*q2(3);
qRes(3) = q1(1)*q2(3) - q1(2)*q2(4) + q1(3)*q2(1) + q1(4)*q2(2);
qRes(4) = q1(1)*q2(4) + q1(2)*q2(3) - q1(3)*q2(2) + q1(4)*q2(1);

== matlab function arducopter/Attitude Controller/input_euler_angle_roll_pitch_euler_rate_yaw()/thrust_heading_rotation_angles()/Yaw error limitation/Yaw limiting and recalculation of attitudeTarget/MATLAB Function1 ==
function qRes = quatMult(q1, q2)
% Quaternion multiplication. Code based on QuaternionT<T>::operator*() in
% quaternion.cpp

qRes = single(zeros(4,1));
qRes(1) = q1(1)*q2(1) - q1(2)*q2(2) - q1(3)*q2(3) - q1(4)*q2(4);
qRes(2) = q1(1)*q2(2) + q1(2)*q2(1) + q1(3)*q2(4) - q1(4)*q2(3);
qRes(3) = q1(1)*q2(3) - q1(2)*q2(4) + q1(3)*q2(1) + q1(4)*q2(2);
qRes(4) = q1(1)*q2(4) + q1(2)*q2(3) - q1(3)*q2(2) + q1(4)*q2(1);

== matlab function arducopter/Attitude Controller/input_euler_angle_roll_pitch_euler_rate_yaw()/update_ang_vel_target_from_att_error()/Calc angular velocity target roll/Square Root Controller ==
function correction_rate = sqrt_controller(err, p, second_ord_lim, dt)
% The square root controller
% Code is taken from sqrt_controller(...) in AC_PosControl.cpp, line 296.

if (second_ord_lim < 0 || second_ord_lim == 0)
   correction_rate = err * p;
elseif (p == 0)
    % P term is zero, but second order limit is positive
    if (err > 0)
        correction_rate = sqrt(single(2.0) * second_ord_lim * err);
    elseif (err < 0)
        correction_rate = sqrt(single(2.0) * second_ord_lim * -err);
    else
        correction_rate = single(0.0);
    end
else
    % P term and second order limit are positive, hence have been defined
    linear_dist = second_ord_lim / (p * p);
    % Check if error exceeds linear range of controller gain
    if (err > linear_dist)
        correction_rate = sqrt(single(2.0) * second_ord_lim * ( err - (linear_dist / single(2.0)) ));
    elseif (err < -linear_dist)
        correction_rate = -sqrt(single(2.0) * second_ord_lim * ( -err - (linear_dist / single(2.0)) ));
    else
        % Return linearly amplified correction if error is in linear range
        correction_rate = err * p;
    end
end

% Prevent oscillations by over-shooting the error correction in the last
% time step
if (dt ~= 0)
    correction_rate = max( min(correction_rate, abs(err) / dt), -abs(err) / dt);
end

== matlab function arducopter/Attitude Controller/input_euler_angle_roll_pitch_euler_rate_yaw()/update_ang_vel_target_from_att_error()/Calc angular velocity target pitch/Square Root Controller ==
function correction_rate = sqrt_controller(err, p, second_ord_lim, dt)
% The square root controller
% Code is taken from sqrt_controller(...) in AC_PosControl.cpp, line 296.

if (second_ord_lim < 0 || second_ord_lim == 0)
   correction_rate = err * p;
elseif (p == 0)
    % P term is zero, but second order limit is positive
    if (err > 0)
        correction_rate = sqrt(single(2.0) * second_ord_lim * err);
    elseif (err < 0)
        correction_rate = sqrt(single(2.0) * second_ord_lim * -err);
    else
        correction_rate = single(0.0);
    end
else
    % P term and second order limit are positive, hence have been defined
    linear_dist = second_ord_lim / (p * p);
    % Check if error exceeds linear range of controller gain
    if (err > linear_dist)
        correction_rate = sqrt(single(2.0) * second_ord_lim * ( err - (linear_dist / single(2.0)) ));
    elseif (err < -linear_dist)
        correction_rate = -sqrt(single(2.0) * second_ord_lim * ( -err - (linear_dist / single(2.0)) ));
    else
        % Return linearly amplified correction if error is in linear range
        correction_rate = err * p;
    end
end

% Prevent oscillations by over-shooting the error correction in the last
% time step
if (dt ~= 0)
    correction_rate = max( min(correction_rate, abs(err) / dt), -abs(err) / dt);
end

== matlab function arducopter/Attitude Controller/input_euler_angle_roll_pitch_euler_rate_yaw()/update_ang_vel_target_from_att_error()/Calc angular velocity target yaw/Square Root Controller ==
function correction_rate = sqrt_controller(err, p, second_ord_lim, dt)
% The square root controller
% Code is taken from sqrt_controller(...) in AC_PosControl.cpp, line 296.

if (second_ord_lim < 0 || second_ord_lim == 0)
   correction_rate = err * p;
elseif (p == 0)
    % P term is zero, but second order limit is positive
    if (err > 0)
        correction_rate = sqrt(single(2.0) * second_ord_lim * err);
    elseif (err < 0)
        correction_rate = sqrt(single(2.0) * second_ord_lim * -err);
    else
        correction_rate = single(0.0);
    end
else
    % P term and second order limit are positive, hence have been defined
    linear_dist = second_ord_lim / (p * p);
    % Check if error exceeds linear range of controller gain
    if (err > linear_dist)
        correction_rate = sqrt(single(2.0) * second_ord_lim * ( err - (linear_dist / single(2.0)) ));
    elseif (err < -linear_dist)
        correction_rate = -sqrt(single(2.0) * second_ord_lim * ( -err - (linear_dist / single(2.0)) ));
    else
        % Return linearly amplified correction if error is in linear range
        correction_rate = err * p;
    end
end

% Prevent oscillations by over-shooting the error correction in the last
% time step
if (dt ~= 0)
    correction_rate = max( min(correction_rate, abs(err) / dt), -abs(err) / dt);
end

== matlab function arducopter/Attitude Controller/input_euler_angle_roll_pitch_euler_rate_yaw()/MATLAB Function2 ==
function angVelLimited = ang_vel_limit(angVel, angVelRollMax, angVelPitchMax, angVelYawMax)
% Limits angular velocity (rad/s) in body frame
% Code based on AC_AttitudeControl::ang_vel_limit()

angVelLimited = angVel;
if angVelRollMax == 0 || angVelPitchMax == 0
    if angVelRollMax ~= 0
        angVelLimited(1) = max(min(angVel(1), angVelRollMax), -angVelRollMax);
    end
    if angVelPitchMax ~= 0
        angVelLimited(2) = max(min(angVel(2), angVelPitchMax), -angVelPitchMax);
    end
else
    thrustVecAngVel = [angVel(1) / angVelRollMax; angVel(2) / angVelPitchMax];
    thrustVecLen = single(sqrt(thrustVecAngVel(1)^2 + thrustVecAngVel(2)^2));
    if thrustVecLen > 1
        angVelLimited(1) = thrustVecAngVel(1) * angVelRollMax / thrustVecLen;
        angVelLimited(2) = thrustVecAngVel(2) * angVelPitchMax / thrustVecLen;
    end
end
if angVelYawMax ~= 0
    angVelLimited(3) = max(min(angVel(3), angVelYawMax), -angVelYawMax);
end

== matlab function arducopter/Attitude Controller/input_euler_angle_roll_pitch_euler_rate_yaw()/MATLAB Function7 ==
function qInv = invertQuat(q)
% Function inverts the rotation of a quaternion.
% Code based on QuaternionT<T>::inverse(void)
% qInv = [q(1);-q(2);-q(3);-q(4)];
qInv = single(zeros(4,1));
qInv(1) = q(1);
qInv(2) = -q(2);
qInv(3) = -q(3);
qInv(4) = -q(4);

== matlab function arducopter/Throttle/Throttle Calculations/Throttle-Attitude-Mixing/Update Throttle Mix ==
function thrMix = updateThrMix(thrMixDes, thrMixMin, thrMixMax, dt)
% The function represents the update_throttle_rpy_mix() function in
% AC_AttitudeControl_Multi.cpp
% The function slowly moves rpy_mix to rpy_mix_des which represents the
% desired mix between hover and thrust throttle.
global thrMixAct

if thrMixAct < thrMixDes
    thrMix = thrMixAct + min(2 * dt, thrMixDes - thrMixAct);
elseif thrMixAct > thrMixDes
    thrMix = thrMixAct - min(0.5 * dt, thrMixAct - thrMixDes);
else   % Added else statement due to compiler error for uninitialized output
    thrMix = thrMixAct;
end

thrMix = max( min( thrMix, thrMixMax), thrMixMin );

== matlab function arducopter/Attitude Controller/input_euler_angle_roll_pitch_euler_rate_yaw()/MATLAB Function11 ==
function qRes = quatMult(q1, q2)
% Quaternion multiplication. Code based on QuaternionT<T>::operator*() in
% quaternion.cpp

qRes = single(zeros(4,1));
qRes(1) = q1(1)*q2(1) - q1(2)*q2(2) - q1(3)*q2(3) - q1(4)*q2(4);
qRes(2) = q1(1)*q2(2) + q1(2)*q2(1) + q1(3)*q2(4) - q1(4)*q2(3);
qRes(3) = q1(1)*q2(3) - q1(2)*q2(4) + q1(3)*q2(1) + q1(4)*q2(2);
qRes(4) = q1(1)*q2(4) + q1(2)*q2(3) - q1(3)*q2(2) + q1(4)*q2(1);

== matlab function arducopter/Attitude Controller/input_euler_angle_roll_pitch_euler_rate_yaw()/MATLAB Function4 ==
function vecRot = rotateByQuat(q, vec)
% Function rotates vector vec by quaternion q. Equivalent to converting the
% input quaternion to a rotation matrix and then multiplying it by the
% vector. This uses the formula
%
%    v2 = v1 + 2 q1 * qv x v1 + 2 qv x qv x v1
%
% where "x" is the cross product (explicitly inlined for performance below), 
% "q1" is the scalar part and "qv" is the vector part of this quaternion
% Code based on Vector3<T> QuaternionT<T>::operator*()

vecRot = vec;

% Compute and cache "qv x v1"
uv = [q(3) * vec(3) - q(4) * vec(2); q(4) * vec(1) - q(2) * vec(3); q(2) * vec(2) - q(3) * vec(1)];

uv(1) = uv(1) + uv(1);
uv(2) = uv(2) + uv(2);
uv(3) = uv(3) + uv(3);
vecRot(1) = vecRot(1) + q(1) * uv(1) + q(3) * uv(3) - q(4) * uv(2);
vecRot(2) = vecRot(2) + q(1) * uv(2) + q(4) * uv(1) - q(2) * uv(3);
vecRot(3) = vecRot(3) + q(1) * uv(3) + q(2) * uv(2) - q(3) * uv(1);

== matlab function arducopter/Attitude Controller/input_euler_angle_roll_pitch_euler_rate_yaw()/Add feedforward to angVelBody/MATLAB Function ==
function [angVelBodyNew, feedforwardScaler] = addFeedforwardToTargetAngVel(angVelBodyFeedforward, angVelBodyIn, thrustErrorAngle, yawRateAct, maxThrustErrorAngle4YawCorr)
% Function smoothly adds feedforward angular velocity and yaw input to
% target angular velocity.
% Code based on AC_AttitudeControl::attitude_controller_run_quat()

angVelBodyNew = angVelBodyIn;

feedforwardScaler = single(1);
if thrustErrorAngle > 2 * maxThrustErrorAngle4YawCorr
    % thrustErrorAngle too large. Set target yaw rate to actual rate. Do not
    % add feedforward.
    angVelBodyNew(3) = yawRateAct;
elseif thrustErrorAngle > maxThrustErrorAngle4YawCorr
    % thrustErrorAngle still large. Add feedforward values smoothly.
    feedforwardScaler = 1 - (thrustErrorAngle - maxThrustErrorAngle4YawCorr) / maxThrustErrorAngle4YawCorr;
    angVelBodyNew(1) = angVelBodyNew(1) + angVelBodyFeedforward(1) * feedforwardScaler;
    angVelBodyNew(2) = angVelBodyNew(2) + angVelBodyFeedforward(2) * feedforwardScaler;
    angVelBodyNew(3) = angVelBodyNew(3) + angVelBodyFeedforward(3);
    angVelBodyNew(3) = yawRateAct * (1 - feedforwardScaler) + angVelBodyNew(3) * feedforwardScaler;
else
    % thrustErrorAngle small enough to add feedforward values to target
    % angular rates of controller without smoothing.
    angVelBodyNew = angVelBodyNew + angVelBodyFeedforward;
end

== matlab function arducopter/Attitude Controller/input_euler_angle_roll_pitch_euler_rate_yaw()/Update attitudeTarget/MATLAB Function ==
function qNorm = normalizeQuat(q)
% Function to normalze a quaternion. Code based on
% QuaternionT<T>::normalize()

quatLen = single(sqrt(q(1)^2 + q(2)^2 + q(3)^2 + q(4)^2));
if quatLen ~= 0
    qNorm = q ./ quatLen;
else
    qNorm = q;
end
